simulink model "indi_controller_tuning"  (R2024b)
settings: Solver=FixedStepAuto  StartTime=0.0  StopTime=inf  FixedStep=0.001  RelTol=1e-3
undefined symbols (not defined in the file): dirty_derivative, drawaircraft, drawaircraft2, dspblkCoreblockFVToolHelper, force_moment, gcbh, INDI, MAV, position_rhombus, reference_model, sample_time, SIM
libraries: slpidlib x12
(part 1 of 2)
settings Model: Creator=SJ  LastModifiedBy=SJ

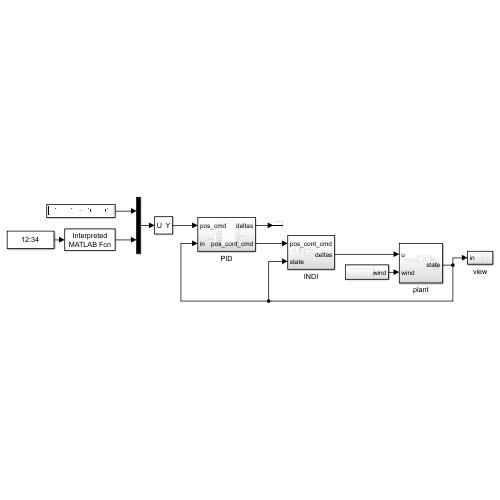
[thumbnail: Simulink's stored preview of the top-level diagram]
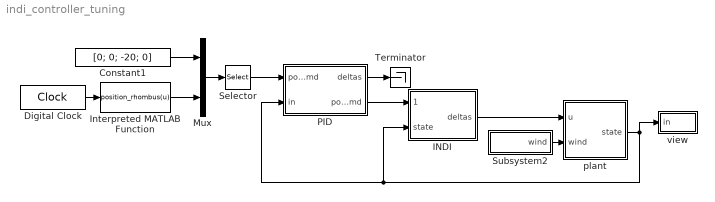
== system indi_controller_tuning ==
  Constant1 : Constant  Value=[0; 0; -20; 0]
  Digital Clock : DigitalClock  SampleTime=0.001
  INDI : Subsystem
  Interpreted MATLAB Function : MATLABFcn  MATLABFcn=position_rhombus(u)  OutputDimensions=4
  Mux : Mux  Inputs=2
  PID : Subsystem
  Selector : Selector  InputPortWidth=8  IndexOptions=Index vector (dialog)  Indices=[5:8]  OutputSizes=1
  Subsystem2 : Subsystem
  Terminator : Terminator
  plant : Subsystem
  view : Subsystem
  wires:
  Subsystem2/1(wind) -> plant/2(wind)
  plant/1(state) -> view/1(in), INDI/2(state), PID/2(in)
  Digital Clock/1 -> Interpreted MATLAB Function/1
  Constant1/1 -> Mux/1
  PID/1(deltas) -> Terminator/1
  INDI/1(deltas) -> plant/1(u)
  PID/2(pos_cont_cmd) -> INDI/1(pos_cont_cmd)
  Mux/1 -> Selector/1
  Selector/1 -> PID/1(pos_cmd)
  Interpreted MATLAB Function/1 -> Mux/2

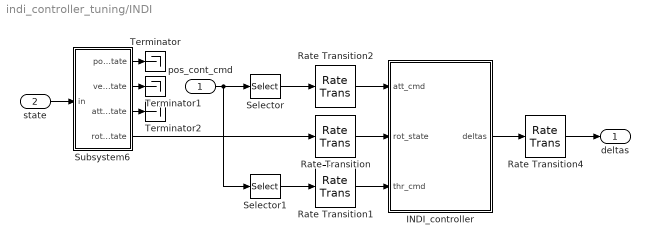
== system indi_controller_tuning/INDI ==
  pos_cont_cmd : Inport
  state : Inport  Port=2
  INDI_controller : Subsystem  TreatAsAtomicUnit=on  SystemSampleTime=sample_time
  Rate Transition : RateTransition  OutPortSampleTime=sample_time
  Rate Transition1 : RateTransition  OutPortSampleTime=sample_time
  Rate Transition2 : RateTransition  OutPortSampleTime=sample_time
  Rate Transition4 : RateTransition
  Selector : Selector  InputPortWidth=4  IndexOptions=Index vector (dialog)  Indices=[1:3]  OutputSizes=1
  Selector1 : Selector  InputPortWidth=4  IndexOptions=Index vector (dialog)  Indices=[4]  OutputSizes=1
  Subsystem6 : Subsystem
  Terminator : Terminator
  Terminator1 : Terminator
  Terminator2 : Terminator
  deltas : Outport
  wires:
  Rate Transition/1 -> INDI_controller/2(rot_state)
  Subsystem6/4(rot_state) -> Rate Transition/1
  Rate Transition1/1 -> INDI_controller/3(thr_cmd)
  INDI_controller/1(deltas) -> Rate Transition4/1
  Rate Transition4/1 -> deltas/1
  Rate Transition2/1 -> INDI_controller/1(att_cmd)
  Selector1/1 -> Rate Transition1/1
  pos_cont_cmd/1 -> Selector1/1, Selector/1
  state/1 -> Subsystem6/1(in)
  Selector/1 -> Rate Transition2/1
  Subsystem6/1(pos_state) -> Terminator/1
  Subsystem6/2(vel_state) -> Terminator1/1
  Subsystem6/3(att_state) -> Terminator2/1

== system indi_controller_tuning/PID ==
  pos_cmd : Inport
  in : Inport  Port=2
  Demux : Demux
  Mux : Mux
  PID_Controller : Subsystem
  Subsystem6 : Subsystem
  deltas : Outport
  pos_cont_cmd : Outport  Port=2
  wires:
  in/1 -> Subsystem6/1(in)
  Demux/4 -> Mux/3, PID_Controller/4(yaw_cmd)
  Demux/1 -> PID_Controller/1(px_cmd)
  Demux/2 -> PID_Controller/2(py_cmd)
  Demux/3 -> PID_Controller/3(pd_cmd)
  Subsystem6/1(pos_state) -> PID_Controller/5(pos_state)
  Subsystem6/2(vel_state) -> PID_Controller/6(vel_state)
  Subsystem6/3(att_state) -> PID_Controller/7(att_state)
  Subsystem6/4(rot_state) -> PID_Controller/8(rot_state)
  PID_Controller/1(deltas) -> deltas/1
  PID_Controller/2(phi_cmd) -> Mux/1
  PID_Controller/3(theta_cmd) -> Mux/2
  PID_Controller/4(thr_cmd) -> Mux/4
  pos_cmd/1 -> Demux/1
  Mux/1 -> pos_cont_cmd/1

== system indi_controller_tuning/Subsystem2 ==
  Constant16 : Constant  Value=[SIM.wind.wn_s; SIM.wind.we_s; SIM.wind.wd_s]
  Constant17 : Constant  Value=[0; 0; 0]
  Mux1 : Mux  Inputs=2
  wind : Outport
  wires:
  Constant16/1 -> Mux1/1
  Mux1/1 -> wind/1  "wind"
  Constant17/1 -> Mux1/2

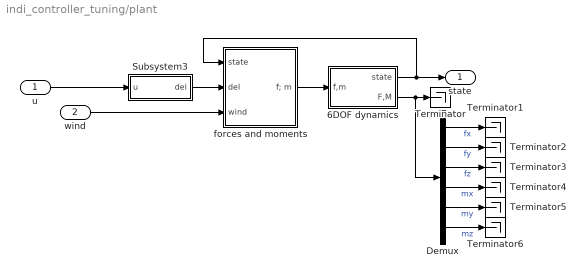
== system indi_controller_tuning/plant ==
  u : Inport
  wind : Inport  Port=2
  6DOF dynamics : Subsystem
  Demux : Demux  Outputs=6
  Subsystem3 : Subsystem
  Terminator{,1..6} (7 alike) : Terminator
  forces and moments : Subsystem
  state : Outport
  wires:
  wind/1 -> forces and moments/3(wind)
  6DOF dynamics/2(F,M) -> Demux/1, Terminator/1
  6DOF dynamics/1(state) -> forces and moments/1(state), state/1
  forces and moments/1(f; m) -> 6DOF dynamics/1(f,m)
  Subsystem3/1(del) -> forces and moments/2(del)
  Demux/1 -> Terminator1/1  "fx"
  Demux/2 -> Terminator2/1  "fy"
  Demux/3 -> Terminator3/1  "fz"
  Demux/4 -> Terminator4/1  "mx"
  Demux/5 -> Terminator5/1  "my"
  Demux/6 -> Terminator6/1  "mz"
  u/1 -> Subsystem3/1(u)

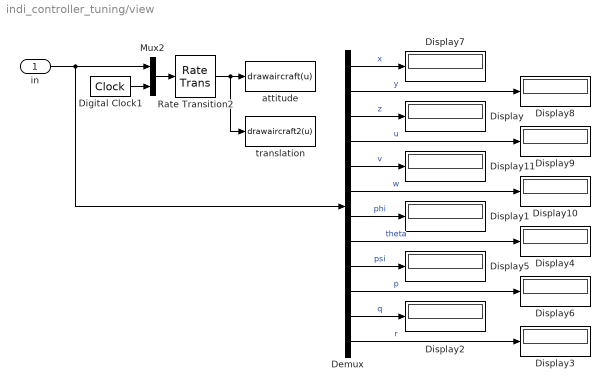
== system indi_controller_tuning/view ==
  in : Inport
  Demux : Demux  Outputs=12
  Digital Clock1 : DigitalClock  SampleTime=0.005
  Display{,1..11} (12 alike) : Display
  Mux2 : Mux  Inputs=2
  Rate Transition2 : RateTransition  OutPortSampleTime=0.1
  attitude : MATLABFcn  MATLABFcn=drawaircraft(u)  OutputDimensions=0
  translation : MATLABFcn  MATLABFcn=drawaircraft2(u)  OutputDimensions=0
  wires:
  Rate Transition2/1 -> translation/1, attitude/1
  Digital Clock1/1 -> Mux2/2
  Mux2/1 -> Rate Transition2/1
  in/1 -> Demux/1, Mux2/1
  Demux/3 -> Display/1  "z"
  Demux/11 -> Display2/1  "q"
  Demux/12 -> Display3/1  "r"
  Demux/8 -> Display4/1  "theta"
  Demux/9 -> Display5/1  "psi"
  Demux/10 -> Display6/1  "p"
  Demux/7 -> Display1/1  "phi"
  Demux/2 -> Display8/1  "y"
  Demux/1 -> Display7/1  "x"
  Demux/4 -> Display9/1  "u"
  Demux/6 -> Display10/1  "w"
  Demux/5 -> Display11/1  "v"

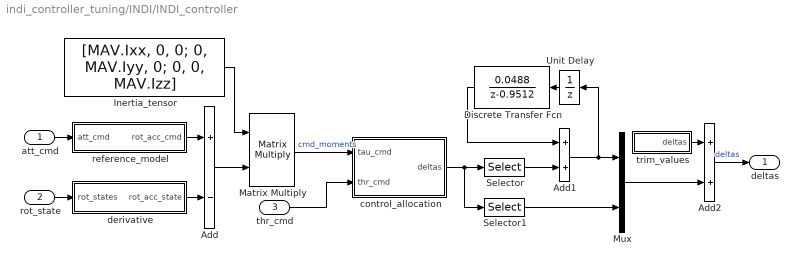
== system indi_controller_tuning/INDI/INDI_controller ==
  att_cmd : Inport  OutDataTypeStr=double  PortDimensions=3
  rot_state : Inport  Port=2  OutDataTypeStr=double  PortDimensions=3
  thr_cmd : Inport  Port=3
  Add : Sum  Inputs=+-
  Add1 : Sum
  Add2 : Sum
  Discrete Transfer Fcn : DiscreteTransferFcn  LoadFcn=dspblkCoreblockFVToolHelper(gcbh,'load');  Numerator=[0.0488]  Denominator=[1 -0.9512]  InitialStates=[0;0;0;0]
      settings: CopyFcn=dspblkCoreblockFVToolHelper(gcbh,'copy');  DeleteFcn=dspblkCoreblockFVToolHelper(gcbh,'close');  ModelCloseFcn=dspblkCoreblockFVToolHelper(gcbh,'close');  PreSaveFcn=dspblkCoreblockFVToolHelper(gcbh,'presave');  PostSaveFcn=dspblkCoreblockFVToolHelper(gcbh,'postsave');  CloseFcn=dspblkCoreblockFVToolHelper(gcbh,'close');
  Inertia_tensor : Constant  Value=[MAV.Ixx, 0, 0; 0, MAV.Iyy, 0; 0, 0, MAV.Izz]
  Matrix Multiply : Product  Multiplication=Matrix(*)
  Mux : Mux  Inputs=2
  Selector : Selector  InputPortWidth=5  IndexOptions=Index vector (dialog)  Indices=[1:4]  OutputSizes=1
  Selector1 : Selector  InputPortWidth=5  IndexOptions=Index vector (dialog)  Indices=[5]  OutputSizes=1
  Unit Delay : UnitDelay  InitialCondition=[0;0;0;0]  SampleTime=sample_time  HasFrameUpgradeWarning=on
  control_allocation : Subsystem
  derivative : Subsystem
  reference_model : Subsystem
  trim_values : Subsystem
  deltas : Outport  OutDataTypeStr=double  PortDimensions=5  SampleTime=[0.0050000000000000001,0]
  wires:
  Matrix Multiply/1 -> control_allocation/1(tau_cmd)  "cmd_moments"
  Discrete Transfer Fcn/1 -> Add1/1
  control_allocation/1(deltas) -> Selector/1, Selector1/1
  Unit Delay/1 -> Discrete Transfer Fcn/1
  Inertia_tensor/1 -> Matrix Multiply/1
  Selector/1 -> Add1/2
  Selector1/1 -> Mux/2
  Mux/1 -> Add2/2
  Add/1 -> Matrix Multiply/2
  thr_cmd/1 -> control_allocation/2(thr_cmd)
  Add1/1 -> Mux/1, Unit Delay/1
  att_cmd/1 -> reference_model/1(att_cmd)
  reference_model/1(rot_acc_cmd) -> Add/1
  rot_state/1 -> derivative/1(rot_states)
  derivative/1(rot_acc_state) -> Add/2
  Add2/1 -> deltas/1  "deltas"
  trim_values/1(deltas) -> Add2/1

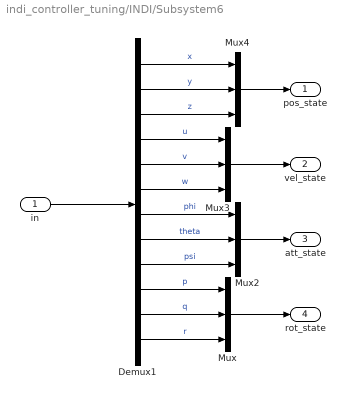
== system indi_controller_tuning/INDI/Subsystem6 ==
  in : Inport
  Demux1 : Demux  Outputs=12
  Mux{,2..4} (4 alike) : Mux  Inputs=3
  pos_state : Outport
  vel_state : Outport  Port=2
  att_state : Outport  Port=3
  rot_state : Outport  Port=4
  wires:
  Mux/1 -> rot_state/1
  Demux1/5 -> Mux3/2  "v"
  Demux1/10 -> Mux/1  "p"
  Demux1/4 -> Mux3/1  "u"
  Demux1/6 -> Mux3/3  "w"
  Demux1/11 -> Mux/2  "q"
  Demux1/7 -> Mux2/1  "phi"
  Demux1/12 -> Mux/3  "r"
  Demux1/8 -> Mux2/2  "theta"
  Demux1/9 -> Mux2/3  "psi"
  Demux1/3 -> Mux4/3  "z"
  Demux1/2 -> Mux4/2  "y"
  Demux1/1 -> Mux4/1  "x"
  Mux2/1 -> att_state/1
  in/1 -> Demux1/1
  Mux3/1 -> vel_state/1
  Mux4/1 -> pos_state/1

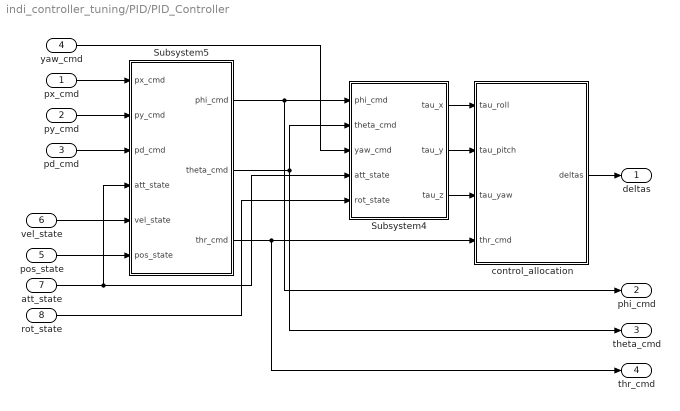
== system indi_controller_tuning/PID/PID_Controller ==
  px_cmd : Inport
  py_cmd : Inport  Port=2
  pd_cmd : Inport  Port=3
  yaw_cmd : Inport  Port=4
  pos_state : Inport  Port=5
  vel_state : Inport  Port=6
  att_state : Inport  Port=7
  rot_state : Inport  Port=8
  Subsystem4 : Subsystem
  Subsystem5 : Subsystem
  control_allocation : Subsystem
  deltas : Outport
  phi_cmd : Outport  Port=2
  theta_cmd : Outport  Port=3
  thr_cmd : Outport  Port=4
  wires:
  Subsystem5/3(thr_cmd) -> thr_cmd/1, control_allocation/4(thr_cmd)
  pos_state/1 -> Subsystem5/6(pos_state)
  Subsystem5/1(phi_cmd) -> phi_cmd/1, Subsystem4/1(phi_cmd)
  Subsystem4/2(tau_y) -> control_allocation/2(tau_pitch)
  att_state/1 -> Subsystem5/4(att_state), Subsystem4/4(att_state)
  px_cmd/1 -> Subsystem5/1(px_cmd)
  Subsystem5/2(theta_cmd) -> theta_cmd/1, Subsystem4/2(theta_cmd)
  Subsystem4/3(tau_z) -> control_allocation/3(tau_yaw)
  Subsystem4/1(tau_x) -> control_allocation/1(tau_roll)
  py_cmd/1 -> Subsystem5/2(py_cmd)
  pd_cmd/1 -> Subsystem5/3(pd_cmd)
  control_allocation/1(deltas) -> deltas/1
  rot_state/1 -> Subsystem4/5(rot_state)
  vel_state/1 -> Subsystem5/5(vel_state)
  yaw_cmd/1 -> Subsystem4/3(yaw_cmd)

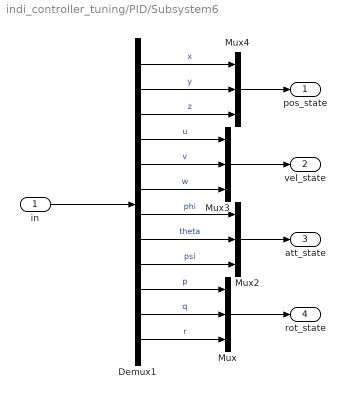
== system indi_controller_tuning/PID/Subsystem6 ==
  in : Inport
  Demux1 : Demux  Outputs=12
  Mux{,2..4} (4 alike) : Mux  Inputs=3
  pos_state : Outport
  vel_state : Outport  Port=2
  att_state : Outport  Port=3
  rot_state : Outport  Port=4
  wires:
  Mux/1 -> rot_state/1
  Demux1/5 -> Mux3/2  "v"
  Demux1/10 -> Mux/1  "p"
  Demux1/4 -> Mux3/1  "u"
  Demux1/6 -> Mux3/3  "w"
  Demux1/11 -> Mux/2  "q"
  Demux1/7 -> Mux2/1  "phi"
  Demux1/12 -> Mux/3  "r"
  Demux1/8 -> Mux2/2  "theta"
  Demux1/9 -> Mux2/3  "psi"
  Demux1/3 -> Mux4/3  "z"
  Demux1/2 -> Mux4/2  "y"
  Demux1/1 -> Mux4/1  "x"
  Mux2/1 -> att_state/1
  in/1 -> Demux1/1
  Mux3/1 -> vel_state/1
  Mux4/1 -> pos_state/1

== system indi_controller_tuning/plant/6DOF dynamics ==
  f,m : Inport
  S-Function : S-Function  FunctionName=UAVdynamics  Parameters=MAV  SFunctionDeploymentMode=off  EnableBusSupport=off
  state : Outport
  F,M : Outport  Port=2
  wires:
  S-Function/1 -> state/1  "state"
  f,m/1 -> S-Function/1, F,M/1

== system indi_controller_tuning/plant/Subsystem3 ==
  u : Inport
  Demux : Demux  Outputs=5
  Mux3 : Mux  Inputs=5
  Transfer Fcn{,1..3} (4 alike) : TransferFcn  Commented=on  Denominator=[MAV.flap.tc 1]
  Transfer Fcn4 : TransferFcn  Commented=on  Denominator=[MAV.prop.tc 1]
  del : Outport
  wires:
  Mux3/1 -> del/1  "del"
  Demux/1 -> Mux3/1  "del1"
  Demux/2 -> Mux3/2  "del2"
  Demux/4 -> Mux3/4  "del4"
  Demux/3 -> Mux3/3  "del3"
  Demux/5 -> Mux3/5  "delt"
  u/1 -> Demux/1

== system indi_controller_tuning/plant/forces and moments ==
  state : Inport
  del : Inport  Port=2
  wind : Inport  Port=3
  Demux : Demux  Outputs=[6,3]
  Interpreted MATLAB Function1 : MATLABFcn  MATLABFcn=force_moment(u(1:12), u(13:17), u(18:23), MAV)  OutputDimensions=9
  Mux : Mux  Inputs=3
  Terminator : Terminator
  f; m : Outport
  wires:
  Demux/2 -> Terminator/1
  Demux/1 -> f; m/1
  Interpreted MATLAB Function1/1 -> Demux/1
  wind/1 -> Mux/3
  del/1 -> Mux/2
  state/1 -> Mux/1
  Mux/1 -> Interpreted MATLAB Function1/1

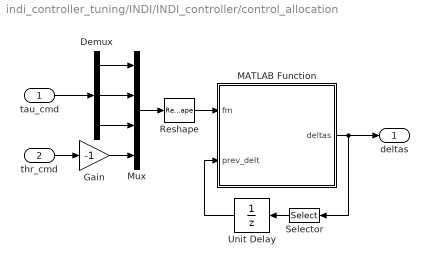
== system indi_controller_tuning/INDI/INDI_controller/control_allocation ==
  tau_cmd : Inport
  thr_cmd : Inport  Port=2
  Demux : Demux  Outputs=3
  Gain : Gain  Gain=-1
  MATLAB Function : MATLAB Function  TreatAsAtomicUnit=on
  Mux : Mux
  Reshape : Reshape  OutputDimensionality=Column vector (2-D)
  Selector : Selector  InputPortWidth=5  IndexOptions=Index vector (dialog)  Indices=[5]  OutputSizes=1
  Unit Delay : UnitDelay  InitialCondition=single(0.724)  SampleTime=sample_time  HasFrameUpgradeWarning=on
  deltas : Outport
  wires:
  Selector/1 -> Unit Delay/1
  tau_cmd/1 -> Demux/1
  Unit Delay/1 -> MATLAB Function/2(prev_delt)
  Demux/3 -> Mux/3
  Mux/1 -> Reshape/1
  thr_cmd/1 -> Gain/1
  Demux/2 -> Mux/2
  Demux/1 -> Mux/1
  MATLAB Function/1(deltas) -> deltas/1, Selector/1
  Reshape/1 -> MATLAB Function/1(fm)
  Gain/1 -> Mux/4

== system indi_controller_tuning/INDI/INDI_controller/derivative ==
  rot_states : Inport
  Data Type Conversion1 : DataTypeConversion  OutDataTypeStr=single  SaturateOnIntegerOverflow=off  RndMeth=Floor
  Interpreted MATLAB Function1 : MATLABFcn  MATLABFcn=dirty_derivative(u(1:3), u(4:9), INDI.derivative.tau, sample_time)  OutputDimensions=6
  Mux : Mux  Inputs=2
  Selector : Selector  InputPortWidth=6  IndexOptions=Index vector (dialog)  Indices=[4:6]  OutputSizes=1
  Unit Delay : UnitDelay  InitialCondition=zeros(6,1)  SampleTime=sample_time  HasFrameUpgradeWarning=on
  rot_acc_state : Outport
  wires:
  Interpreted MATLAB Function1/1 -> Unit Delay/1, Selector/1
  rot_states/1 -> Mux/1
  Data Type Conversion1/1 -> rot_acc_state/1  "rot_acc_state"
  Unit Delay/1 -> Mux/2
  Mux/1 -> Interpreted MATLAB Function1/1
  Selector/1 -> Data Type Conversion1/1

== system indi_controller_tuning/INDI/INDI_controller/reference_model ==
  att_cmd : Inport
  Data Type Conversion : DataTypeConversion  OutDataTypeStr=single  SaturateOnIntegerOverflow=off  RndMeth=Floor
  Mux1 : Mux  Inputs=2
  Selecto r2 : Selector  InputPortWidth=9  IndexOptions=Index vector (dialog)  Indices=[7:9]  OutputSizes=1
  Unit Delay1 : UnitDelay  InitialCondition=zeros(9,1)  SampleTime=sample_time  HasFrameUpgradeWarning=on
  reference_model : MATLABFcn  MATLABFcn=reference_model(u(1:3), u(4:12), INDI.ref_mdl.wn, INDI.ref_mdl.zeta, sample_time)  OutputDimensions=9
  rot_acc_cmd : Outport
  wires:
  reference_model/1 -> Unit Delay1/1, Selecto r2/1
  Mux1/1 -> reference_model/1
  Selecto r2/1 -> Data Type Conversion/1
  Unit Delay1/1 -> Mux1/2
  Data Type Conversion/1 -> rot_acc_cmd/1  "rot_acc_cmd"
  att_cmd/1 -> Mux1/1

== system indi_controller_tuning/INDI/INDI_controller/trim_values ==
  MATLAB Function : MATLAB Function  TreatAsAtomicUnit=on
  Selector2 : Selector  InputPortWidth=5  IndexOptions=Index vector (dialog)  Indices=[5]  OutputSizes=1
  Subsystem1 : Subsystem
  Unit Delay1 : UnitDelay  InitialCondition=single(0.724)  SampleTime=sample_time  HasFrameUpgradeWarning=on
  deltas : Outport
  wires:
  Selector2/1 -> Unit Delay1/1
  MATLAB Function/1(deltas) -> deltas/1, Selector2/1
  Subsystem1/1(cmd) -> MATLAB Function/1(fm)
  Unit Delay1/1 -> MATLAB Function/2(prev_delt)

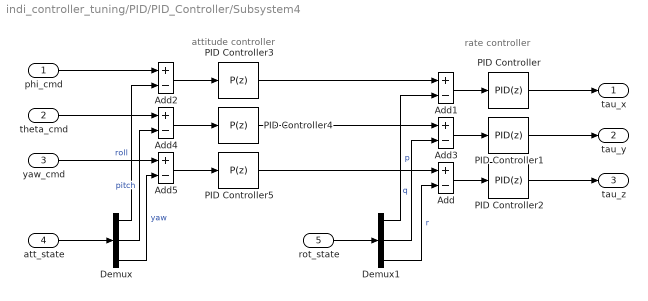
== system indi_controller_tuning/PID/PID_Controller/Subsystem4 ==
  note: rate controller
  note: attitude controller
  phi_cmd : Inport
  theta_cmd : Inport  Port=2
  yaw_cmd : Inport  Port=3
  att_state : Inport  Port=4
  rot_state : Inport  Port=5
  Add{,1..5} (6 alike) : Sum  Inputs=+-
  Demux : Demux  Outputs=3
  Demux1 : Demux  Outputs=3
  PID Controller : slpidlib/PID Controller  Controller=PID  Form=Parallel  TimeDomain=Discrete-time  UseExternalTs=off  SampleTime=sample_time  IntegratorMethod=Forward Euler  FilterMethod=Forward Euler  ControllerParametersSource=internal  P=43.8593962086828  I=273.441461197381  UseKiTs=off  D=0  UseExternalDerivativeSource=off  N=100  UseFilter=on  TunerSelectOption=Transfer Function Based (PID Tuner App)  InitialConditionSource=internal  InitialConditionForIntegrator=0  InitialConditionForFilter=0  DifferentiatorICPrevScaledInput=0  ExternalReset=none  TrackingMode=off  Kt=1  LimitOutput=on  SatLimitsSource=internal  UpperSaturationLimit=1  LowerSaturationLimit=-1  LinearizeAsGain=on  AntiWindupMode=clamping  Kb=1  LimitIntegrator=off  UpperIntegratorSaturationLimit=inf  LowerIntegratorSaturationLimit=-inf  POutMin=[]  POutMax=[]  IOutMin=[]  IOutMax=[]  DOutMin=[]  DOutMax=[]  NOutMin=[]  NOutMax=[]  SumOutMin=[]  SumOutMax=[]  SaturationOutMin=[]  SaturationOutMax=[]  PParamMin=[]  PParamMax=[]  IParamMin=[]  IParamMax=[]  DParamMin=[]  DParamMax=[]  NParamMin=[]  NParamMax=[]  KbParamMin=[]  KbParamMax=[]  KtParamMin=[]  KtParamMax=[]  KbOutMin=[]  KbOutMax=[]  KtOutMin=[]  KtOutMax=[]  IntegratorOutMin=[]  IntegratorOutMax=[]  FilterOutMin=[]  FilterOutMax=[]  SumI1OutMin=[]  SumI1OutMax=[]  SumI2OutMin=[]  SumI2OutMax=[]  SumI3OutMin=[]  SumI3OutMax=[]  SumI4OutMin=[]  SumI4OutMax=[]  SumDOutMin=[]  SumDOutMax=[]  DifferentiatorOutMin=[]  DifferentiatorOutMax=[]  FilterDiffOutCoefMin=[]  FilterDiffOutCoefMax=[]  ReciprocalOutMin=[]  ReciprocalOutMax=[]  SumDenOutMin=[]  SumDenOutMax=[]  SumNumOutMin=[]  SumNumOutMax=[]  DivideOutMin=[]  DivideOutMax=[]  UdiffTsProdOutMin=[]  UdiffTsProdOutMax=[]  NTsProdOutMin=[]  NTsProdOutMax=[]  UintegralTsProdOutMin=[]  UintegralTsProdOutMax=[]  UngainTsProdOutMin=[]  UngainTsProdOutMax=[]  ClampingZeroOutDataTypeStr=Inherit: Inherit via back propagation  ClampingZeroOutMin=[]  ClampingZeroOutMax=[]  FilterDenConstantOutDataTypeStr=Inherit: Inherit via back propagation  FilterDenConstantOutMin=[]  FilterDenConstantOutMax=[]  PCopyOutDataTypeStr=Inherit: Inherit via back propagation  PCopyOutMin=[]  PCopyOutMax=[]  NCopyOutDataTypeStr=Inherit: Inherit via back propagation  NCopyOutMin=[]  NCopyOutMax=[]  IntegratorContinuousStateAttributes=''  IntegratorStateMustResolveToSignalObject=off  IntegratorRTWStateStorageClass=Auto  FilterContinuousStateAttributes=''  FilterStateMustResolveToSignalObject=off  FilterRTWStateStorageClass=Auto  ParallelPVariant=InternalParameters  IdealPVariant=Disabled  IVariant=InternalParameters  DVariant=InternalParameters  IntegratorVariant=Discrete  SatVariant=Enabled  AWVariant=DiscClampingParallel  PCopyVariant=Disabled  TRVariant=Disabled  FdbkBlocksVariant=Forward  IdealPFdbkVariant=Disabled  SatFdbkVariant=Disabled  DerivativeFilterVariant=ForwardEulerFilter  NVariant=InternalParameters  NCopyVariant=Disabled  FilterICVariant=InternalICsFilter  IntegratorICVariant=InternalICs  ExternalResetVariant=Disabled  TRSumVariant=Passthrough  SumFdbkVariant=Disabled  SumVariant=Sum_PID  TsampFilterVariant=InternalTs  TsampNgainVariant=Passthrough  TsampIntegralVariant=Disabled_SignalSpec  ExternalSaturationOutDataTypeStr=Inherit: Same as second input  DerivativeSourceVariant=ErrorSignal  PreIntVariant=InternalPreInt
  PID Controller1 : slpidlib/PID Controller  Controller=PID  Form=Parallel  TimeDomain=Discrete-time  UseExternalTs=off  SampleTime=sample_time  IntegratorMethod=Forward Euler  FilterMethod=Forward Euler  ControllerParametersSource=internal  P=10.8322386798583  I=19.1330051709658  UseKiTs=off  D=0.205716499185363  UseExternalDerivativeSource=off  N=36.46824066771  UseFilter=on  TunerSelectOption=Transfer Function Based (PID Tuner App)  InitialConditionSource=internal  InitialConditionForIntegrator=0  InitialConditionForFilter=0  DifferentiatorICPrevScaledInput=0  ExternalReset=none  TrackingMode=off  Kt=1  LimitOutput=on  SatLimitsSource=internal  UpperSaturationLimit=1  LowerSaturationLimit=-1  LinearizeAsGain=on  AntiWindupMode=clamping  Kb=1  LimitIntegrator=off  UpperIntegratorSaturationLimit=inf  LowerIntegratorSaturationLimit=-inf  POutMin=[]  POutMax=[]  IOutMin=[]  IOutMax=[]  DOutMin=[]  DOutMax=[]  NOutMin=[]  NOutMax=[]  SumOutMin=[]  SumOutMax=[]  SaturationOutMin=[]  SaturationOutMax=[]  PParamMin=[]  PParamMax=[]  IParamMin=[]  IParamMax=[]  DParamMin=[]  DParamMax=[]  NParamMin=[]  NParamMax=[]  KbParamMin=[]  KbParamMax=[]  KtParamMin=[]  KtParamMax=[]  KbOutMin=[]  KbOutMax=[]  KtOutMin=[]  KtOutMax=[]  IntegratorOutMin=[]  IntegratorOutMax=[]  FilterOutMin=[]  FilterOutMax=[]  SumI1OutMin=[]  SumI1OutMax=[]  SumI2OutMin=[]  SumI2OutMax=[]  SumI3OutMin=[]  SumI3OutMax=[]  SumI4OutMin=[]  SumI4OutMax=[]  SumDOutMin=[]  SumDOutMax=[]  DifferentiatorOutMin=[]  DifferentiatorOutMax=[]  FilterDiffOutCoefMin=[]  FilterDiffOutCoefMax=[]  ReciprocalOutMin=[]  ReciprocalOutMax=[]  SumDenOutMin=[]  SumDenOutMax=[]  SumNumOutMin=[]  SumNumOutMax=[]  DivideOutMin=[]  DivideOutMax=[]  UdiffTsProdOutMin=[]  UdiffTsProdOutMax=[]  NTsProdOutMin=[]  NTsProdOutMax=[]  UintegralTsProdOutMin=[]  UintegralTsProdOutMax=[]  UngainTsProdOutMin=[]  UngainTsProdOutMax=[]  ClampingZeroOutDataTypeStr=Inherit: Inherit via back propagation  ClampingZeroOutMin=[]  ClampingZeroOutMax=[]  FilterDenConstantOutDataTypeStr=Inherit: Inherit via back propagation  FilterDenConstantOutMin=[]  FilterDenConstantOutMax=[]  PCopyOutDataTypeStr=Inherit: Inherit via back propagation  PCopyOutMin=[]  PCopyOutMax=[]  NCopyOutDataTypeStr=Inherit: Inherit via back propagation  NCopyOutMin=[]  NCopyOutMax=[]  IntegratorContinuousStateAttributes=''  IntegratorStateMustResolveToSignalObject=off  IntegratorRTWStateStorageClass=Auto  FilterContinuousStateAttributes=''  FilterStateMustResolveToSignalObject=off  FilterRTWStateStorageClass=Auto  ParallelPVariant=InternalParameters  IdealPVariant=Disabled  IVariant=InternalParameters  DVariant=InternalParameters  IntegratorVariant=Discrete  SatVariant=Enabled  AWVariant=DiscClampingParallel  PCopyVariant=Disabled  TRVariant=Disabled  FdbkBlocksVariant=Forward  IdealPFdbkVariant=Disabled  SatFdbkVariant=Disabled  DerivativeFilterVariant=ForwardEulerFilter  NVariant=InternalParameters  NCopyVariant=Disabled  FilterICVariant=InternalICsFilter  IntegratorICVariant=InternalICs  ExternalResetVariant=Disabled  TRSumVariant=Passthrough  SumFdbkVariant=Disabled  SumVariant=Sum_PID  TsampFilterVariant=InternalTs  TsampNgainVariant=Passthrough  TsampIntegralVariant=Disabled_SignalSpec  ExternalSaturationOutDataTypeStr=Inherit: Same as second input  DerivativeSourceVariant=ErrorSignal  PreIntVariant=InternalPreInt
  PID Controller2 : slpidlib/PID Controller  Controller=PID  Form=Parallel  TimeDomain=Discrete-time  UseExternalTs=off  SampleTime=sample_time  IntegratorMethod=Forward Euler  FilterMethod=Forward Euler  ControllerParametersSource=internal  P=16.7530299130484  I=15.5635829644252  UseKiTs=off  D=-0.0149856418026023  UseExternalDerivativeSource=off  N=294.413298802986  UseFilter=on  TunerSelectOption=Transfer Function Based (PID Tuner App)  InitialConditionSource=internal  InitialConditionForIntegrator=0  InitialConditionForFilter=0  DifferentiatorICPrevScaledInput=0  ExternalReset=none  TrackingMode=off  Kt=1  LimitOutput=on  SatLimitsSource=internal  UpperSaturationLimit=1  LowerSaturationLimit=-1  LinearizeAsGain=off  AntiWindupMode=clamping  Kb=1  LimitIntegrator=off  UpperIntegratorSaturationLimit=inf  LowerIntegratorSaturationLimit=-inf  POutMin=[]  POutMax=[]  IOutMin=[]  IOutMax=[]  DOutMin=[]  DOutMax=[]  NOutMin=[]  NOutMax=[]  SumOutMin=[]  SumOutMax=[]  SaturationOutMin=[]  SaturationOutMax=[]  PParamMin=[]  PParamMax=[]  IParamMin=[]  IParamMax=[]  DParamMin=[]  DParamMax=[]  NParamMin=[]  NParamMax=[]  KbParamMin=[]  KbParamMax=[]  KtParamMin=[]  KtParamMax=[]  KbOutMin=[]  KbOutMax=[]  KtOutMin=[]  KtOutMax=[]  IntegratorOutMin=[]  IntegratorOutMax=[]  FilterOutMin=[]  FilterOutMax=[]  SumI1OutMin=[]  SumI1OutMax=[]  SumI2OutMin=[]  SumI2OutMax=[]  SumI3OutMin=[]  SumI3OutMax=[]  SumI4OutMin=[]  SumI4OutMax=[]  SumDOutMin=[]  SumDOutMax=[]  DifferentiatorOutMin=[]  DifferentiatorOutMax=[]  FilterDiffOutCoefMin=[]  FilterDiffOutCoefMax=[]  ReciprocalOutMin=[]  ReciprocalOutMax=[]  SumDenOutMin=[]  SumDenOutMax=[]  SumNumOutMin=[]  SumNumOutMax=[]  DivideOutMin=[]  DivideOutMax=[]  UdiffTsProdOutMin=[]  UdiffTsProdOutMax=[]  NTsProdOutMin=[]  NTsProdOutMax=[]  UintegralTsProdOutMin=[]  UintegralTsProdOutMax=[]  UngainTsProdOutMin=[]  UngainTsProdOutMax=[]  ClampingZeroOutDataTypeStr=Inherit: Inherit via back propagation  ClampingZeroOutMin=[]  ClampingZeroOutMax=[]  FilterDenConstantOutDataTypeStr=Inherit: Inherit via back propagation  FilterDenConstantOutMin=[]  FilterDenConstantOutMax=[]  PCopyOutDataTypeStr=Inherit: Inherit via back propagation  PCopyOutMin=[]  PCopyOutMax=[]  NCopyOutDataTypeStr=Inherit: Inherit via back propagation  NCopyOutMin=[]  NCopyOutMax=[]  IntegratorContinuousStateAttributes=''  IntegratorStateMustResolveToSignalObject=off  IntegratorRTWStateStorageClass=Auto  FilterContinuousStateAttributes=''  FilterStateMustResolveToSignalObject=off  FilterRTWStateStorageClass=Auto  ParallelPVariant=InternalParameters  IdealPVariant=Disabled  IVariant=InternalParameters  DVariant=InternalParameters  IntegratorVariant=Discrete  SatVariant=Enabled  AWVariant=DiscClampingParallel  PCopyVariant=Disabled  TRVariant=Disabled  FdbkBlocksVariant=Forward  IdealPFdbkVariant=Disabled  SatFdbkVariant=Disabled  DerivativeFilterVariant=ForwardEulerFilter  NVariant=InternalParameters  NCopyVariant=Disabled  FilterICVariant=InternalICsFilter  IntegratorICVariant=InternalICs  ExternalResetVariant=Disabled  TRSumVariant=Passthrough  SumFdbkVariant=Disabled  SumVariant=Sum_PID  TsampFilterVariant=InternalTs  TsampNgainVariant=Passthrough  TsampIntegralVariant=Disabled_SignalSpec  ExternalSaturationOutDataTypeStr=Inherit: Same as second input  DerivativeSourceVariant=ErrorSignal  PreIntVariant=InternalPreInt
  PID Controller3 : slpidlib/PID Controller  Controller=P  Form=Parallel  TimeDomain=Discrete-time  UseExternalTs=off  SampleTime=sample_time  IntegratorMethod=Forward Euler  FilterMethod=Forward Euler  ControllerParametersSource=internal  P=1.86586797303387  I=1  UseKiTs=off  D=0  UseExternalDerivativeSource=off  N=100  UseFilter=on  TunerSelectOption=Transfer Function Based (PID Tuner App)  InitialConditionSource=internal  InitialConditionForIntegrator=0  InitialConditionForFilter=0  DifferentiatorICPrevScaledInput=0  ExternalReset=none  TrackingMode=off  Kt=1  LimitOutput=on  SatLimitsSource=internal  UpperSaturationLimit=deg2rad(35)  LowerSaturationLimit=-deg2rad(35)  LinearizeAsGain=on  AntiWindupMode=none  Kb=1  LimitIntegrator=off  UpperIntegratorSaturationLimit=inf  LowerIntegratorSaturationLimit=-inf  POutMin=[]  POutMax=[]  IOutMin=[]  IOutMax=[]  DOutMin=[]  DOutMax=[]  NOutMin=[]  NOutMax=[]  SumOutMin=[]  SumOutMax=[]  SaturationOutMin=[]  SaturationOutMax=[]  PParamMin=[]  PParamMax=[]  IParamMin=[]  IParamMax=[]  DParamMin=[]  DParamMax=[]  NParamMin=[]  NParamMax=[]  KbParamMin=[]  KbParamMax=[]  KtParamMin=[]  KtParamMax=[]  KbOutMin=[]  KbOutMax=[]  KtOutMin=[]  KtOutMax=[]  IntegratorOutMin=[]  IntegratorOutMax=[]  FilterOutMin=[]  FilterOutMax=[]  SumI1OutMin=[]  SumI1OutMax=[]  SumI2OutMin=[]  SumI2OutMax=[]  SumI3OutMin=[]  SumI3OutMax=[]  SumI4OutMin=[]  SumI4OutMax=[]  SumDOutMin=[]  SumDOutMax=[]  DifferentiatorOutMin=[]  DifferentiatorOutMax=[]  FilterDiffOutCoefMin=[]  FilterDiffOutCoefMax=[]  ReciprocalOutMin=[]  ReciprocalOutMax=[]  SumDenOutMin=[]  SumDenOutMax=[]  SumNumOutMin=[]  SumNumOutMax=[]  DivideOutMin=[]  DivideOutMax=[]  UdiffTsProdOutMin=[]  UdiffTsProdOutMax=[]  NTsProdOutMin=[]  NTsProdOutMax=[]  UintegralTsProdOutMin=[]  UintegralTsProdOutMax=[]  UngainTsProdOutMin=[]  UngainTsProdOutMax=[]  ClampingZeroOutDataTypeStr=Inherit: Inherit via back propagation  ClampingZeroOutMin=[]  ClampingZeroOutMax=[]  FilterDenConstantOutDataTypeStr=Inherit: Inherit via back propagation  FilterDenConstantOutMin=[]  FilterDenConstantOutMax=[]  PCopyOutDataTypeStr=Inherit: Inherit via back propagation  PCopyOutMin=[]  PCopyOutMax=[]  NCopyOutDataTypeStr=Inherit: Inherit via back propagation  NCopyOutMin=[]  NCopyOutMax=[]  IntegratorContinuousStateAttributes=''  IntegratorStateMustResolveToSignalObject=off  IntegratorRTWStateStorageClass=Auto  FilterContinuousStateAttributes=''  FilterStateMustResolveToSignalObject=off  FilterRTWStateStorageClass=Auto  ParallelPVariant=InternalParameters  IdealPVariant=Disabled  IVariant=Disabled  DVariant=Disabled  IntegratorVariant=Disabled  SatVariant=Enabled  AWVariant=Disabled  PCopyVariant=Disabled  TRVariant=Disabled  FdbkBlocksVariant=Forward  IdealPFdbkVariant=Disabled  SatFdbkVariant=Disabled  DerivativeFilterVariant=Disabled  NVariant=Disabled  NCopyVariant=Disabled_SignalSpec  FilterICVariant=Disabled  IntegratorICVariant=Disabled  ExternalResetVariant=Disabled  TRSumVariant=Passthrough  SumFdbkVariant=Disabled  SumVariant=Passthrough_P  TsampFilterVariant=InternalTs  TsampNgainVariant=Passthrough  TsampIntegralVariant=Disabled_SignalSpec  ExternalSaturationOutDataTypeStr=Inherit: Same as second input  DerivativeSourceVariant=Disabled  PreIntVariant=InternalPreInt
  PID Controller4 : slpidlib/PID Controller  Controller=P  Form=Parallel  TimeDomain=Discrete-time  UseExternalTs=off  SampleTime=sample_time  IntegratorMethod=Forward Euler  FilterMethod=Forward Euler  ControllerParametersSource=internal  P=1.73858414764148  I=1  UseKiTs=off  D=0  UseExternalDerivativeSource=off  N=100  UseFilter=on  TunerSelectOption=Transfer Function Based (PID Tuner App)  InitialConditionSource=internal  InitialConditionForIntegrator=0  InitialConditionForFilter=0  DifferentiatorICPrevScaledInput=0  ExternalReset=none  TrackingMode=off  Kt=1  LimitOutput=on  SatLimitsSource=internal  UpperSaturationLimit=deg2rad(35)  LowerSaturationLimit=-deg2rad(35)  LinearizeAsGain=on  AntiWindupMode=none  Kb=1  LimitIntegrator=off  UpperIntegratorSaturationLimit=inf  LowerIntegratorSaturationLimit=-inf  POutMin=[]  POutMax=[]  IOutMin=[]  IOutMax=[]  DOutMin=[]  DOutMax=[]  NOutMin=[]  NOutMax=[]  SumOutMin=[]  SumOutMax=[]  SaturationOutMin=[]  SaturationOutMax=[]  PParamMin=[]  PParamMax=[]  IParamMin=[]  IParamMax=[]  DParamMin=[]  DParamMax=[]  NParamMin=[]  NParamMax=[]  KbParamMin=[]  KbParamMax=[]  KtParamMin=[]  KtParamMax=[]  KbOutMin=[]  KbOutMax=[]  KtOutMin=[]  KtOutMax=[]  IntegratorOutMin=[]  IntegratorOutMax=[]  FilterOutMin=[]  FilterOutMax=[]  SumI1OutMin=[]  SumI1OutMax=[]  SumI2OutMin=[]  SumI2OutMax=[]  SumI3OutMin=[]  SumI3OutMax=[]  SumI4OutMin=[]  SumI4OutMax=[]  SumDOutMin=[]  SumDOutMax=[]  DifferentiatorOutMin=[]  DifferentiatorOutMax=[]  FilterDiffOutCoefMin=[]  FilterDiffOutCoefMax=[]  ReciprocalOutMin=[]  ReciprocalOutMax=[]  SumDenOutMin=[]  SumDenOutMax=[]  SumNumOutMin=[]  SumNumOutMax=[]  DivideOutMin=[]  DivideOutMax=[]  UdiffTsProdOutMin=[]  UdiffTsProdOutMax=[]  NTsProdOutMin=[]  NTsProdOutMax=[]  UintegralTsProdOutMin=[]  UintegralTsProdOutMax=[]  UngainTsProdOutMin=[]  UngainTsProdOutMax=[]  ClampingZeroOutDataTypeStr=Inherit: Inherit via back propagation  ClampingZeroOutMin=[]  ClampingZeroOutMax=[]  FilterDenConstantOutDataTypeStr=Inherit: Inherit via back propagation  FilterDenConstantOutMin=[]  FilterDenConstantOutMax=[]  PCopyOutDataTypeStr=Inherit: Inherit via back propagation  PCopyOutMin=[]  PCopyOutMax=[]  NCopyOutDataTypeStr=Inherit: Inherit via back propagation  NCopyOutMin=[]  NCopyOutMax=[]  IntegratorContinuousStateAttributes=''  IntegratorStateMustResolveToSignalObject=off  IntegratorRTWStateStorageClass=Auto  FilterContinuousStateAttributes=''  FilterStateMustResolveToSignalObject=off  FilterRTWStateStorageClass=Auto  ParallelPVariant=InternalParameters  IdealPVariant=Disabled  IVariant=Disabled  DVariant=Disabled  IntegratorVariant=Disabled  SatVariant=Enabled  AWVariant=Disabled  PCopyVariant=Disabled  TRVariant=Disabled  FdbkBlocksVariant=Forward  IdealPFdbkVariant=Disabled  SatFdbkVariant=Disabled  DerivativeFilterVariant=Disabled  NVariant=Disabled  NCopyVariant=Disabled_SignalSpec  FilterICVariant=Disabled  IntegratorICVariant=Disabled  ExternalResetVariant=Disabled  TRSumVariant=Passthrough  SumFdbkVariant=Disabled  SumVariant=Passthrough_P  TsampFilterVariant=InternalTs  TsampNgainVariant=Passthrough  TsampIntegralVariant=Disabled_SignalSpec  ExternalSaturationOutDataTypeStr=Inherit: Same as second input  DerivativeSourceVariant=Disabled  PreIntVariant=InternalPreInt
  PID Controller5 : slpidlib/PID Controller  Controller=P  Form=Parallel  TimeDomain=Discrete-time  UseExternalTs=off  SampleTime=sample_time  IntegratorMethod=Forward Euler  FilterMethod=Forward Euler  ControllerParametersSource=internal  P=2.2173105634398  I=27.4498971767803  UseKiTs=off  D=0.361274824568414  UseExternalDerivativeSource=off  N=33.4275914175499  UseFilter=on  TunerSelectOption=Transfer Function Based (PID Tuner App)  InitialConditionSource=internal  InitialConditionForIntegrator=0  InitialConditionForFilter=0  DifferentiatorICPrevScaledInput=0  ExternalReset=none  TrackingMode=off  Kt=1  LimitOutput=on  SatLimitsSource=internal  UpperSaturationLimit=deg2rad(45)  LowerSaturationLimit=-deg2rad(45)  LinearizeAsGain=on  AntiWindupMode=none  Kb=1  LimitIntegrator=off  UpperIntegratorSaturationLimit=inf  LowerIntegratorSaturationLimit=-inf  POutMin=[]  POutMax=[]  IOutMin=[]  IOutMax=[]  DOutMin=[]  DOutMax=[]  NOutMin=[]  NOutMax=[]  SumOutMin=[]  SumOutMax=[]  SaturationOutMin=[]  SaturationOutMax=[]  PParamMin=[]  PParamMax=[]  IParamMin=[]  IParamMax=[]  DParamMin=[]  DParamMax=[]  NParamMin=[]  NParamMax=[]  KbParamMin=[]  KbParamMax=[]  KtParamMin=[]  KtParamMax=[]  KbOutMin=[]  KbOutMax=[]  KtOutMin=[]  KtOutMax=[]  IntegratorOutMin=[]  IntegratorOutMax=[]  FilterOutMin=[]  FilterOutMax=[]  SumI1OutMin=[]  SumI1OutMax=[]  SumI2OutMin=[]  SumI2OutMax=[]  SumI3OutMin=[]  SumI3OutMax=[]  SumI4OutMin=[]  SumI4OutMax=[]  SumDOutMin=[]  SumDOutMax=[]  DifferentiatorOutMin=[]  DifferentiatorOutMax=[]  FilterDiffOutCoefMin=[]  FilterDiffOutCoefMax=[]  ReciprocalOutMin=[]  ReciprocalOutMax=[]  SumDenOutMin=[]  SumDenOutMax=[]  SumNumOutMin=[]  SumNumOutMax=[]  DivideOutMin=[]  DivideOutMax=[]  UdiffTsProdOutMin=[]  UdiffTsProdOutMax=[]  NTsProdOutMin=[]  NTsProdOutMax=[]  UintegralTsProdOutMin=[]  UintegralTsProdOutMax=[]  UngainTsProdOutMin=[]  UngainTsProdOutMax=[]  ClampingZeroOutDataTypeStr=Inherit: Inherit via back propagation  ClampingZeroOutMin=[]  ClampingZeroOutMax=[]  FilterDenConstantOutDataTypeStr=Inherit: Inherit via back propagation  FilterDenConstantOutMin=[]  FilterDenConstantOutMax=[]  PCopyOutDataTypeStr=Inherit: Inherit via back propagation  PCopyOutMin=[]  PCopyOutMax=[]  NCopyOutDataTypeStr=Inherit: Inherit via back propagation  NCopyOutMin=[]  NCopyOutMax=[]  IntegratorContinuousStateAttributes=''  IntegratorStateMustResolveToSignalObject=off  IntegratorRTWStateStorageClass=Auto  FilterContinuousStateAttributes=''  FilterStateMustResolveToSignalObject=off  FilterRTWStateStorageClass=Auto  ParallelPVariant=InternalParameters  IdealPVariant=Disabled  IVariant=Disabled  DVariant=Disabled  IntegratorVariant=Disabled  SatVariant=Enabled  AWVariant=Disabled  PCopyVariant=Disabled  TRVariant=Disabled  FdbkBlocksVariant=Forward  IdealPFdbkVariant=Disabled  SatFdbkVariant=Disabled  DerivativeFilterVariant=Disabled  NVariant=Disabled  NCopyVariant=Disabled_SignalSpec  FilterICVariant=Disabled  IntegratorICVariant=Disabled  ExternalResetVariant=Disabled  TRSumVariant=Passthrough  SumFdbkVariant=Disabled  SumVariant=Passthrough_P  TsampFilterVariant=InternalTs  TsampNgainVariant=Passthrough  TsampIntegralVariant=Disabled_SignalSpec  ExternalSaturationOutDataTypeStr=Inherit: Same as second input  DerivativeSourceVariant=Disabled  PreIntVariant=InternalPreInt
  tau_x : Outport
  tau_y : Outport  Port=2
  tau_z : Outport  Port=3
  wires:
  phi_cmd/1 -> Add2/1
  Add3/1 -> PID Controller1/1
  Add1/1 -> PID Controller/1
  PID Controller/1 -> tau_x/1
  Add4/1 -> PID Controller4/1
  PID Controller4/1 -> Add3/1
  theta_cmd/1 -> Add4/1
  Add2/1 -> PID Controller3/1
  PID Controller1/1 -> tau_y/1
  Demux/1 -> Add2/2  "roll"
  Demux/2 -> Add4/2  "pitch"
  Demux/3 -> Add5/2  "yaw"
  att_state/1 -> Demux/1
  rot_state/1 -> Demux1/1
  Demux1/1 -> Add1/2  "p"
  Demux1/2 -> Add3/2  "q"
  PID Controller5/1 -> Add/1
  PID Controller2/1 -> tau_z/1
  Add5/1 -> PID Controller5/1
  Add/1 -> PID Controller2/1
  Demux1/3 -> Add/2  "r"
  yaw_cmd/1 -> Add5/1
  PID Controller3/1 -> Add1/1
